simulink model "simulink_ODE_solved"  (R2023a)
settings: Solver=ode45  StartTime=0.0  StopTime=3000  RelTol=1e-3
settings Model: Creator=USER  LastModifiedBy=USER

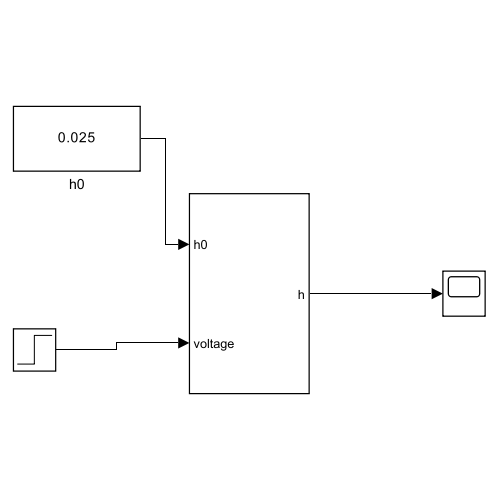
[thumbnail: Simulink's stored preview of the top-level diagram]
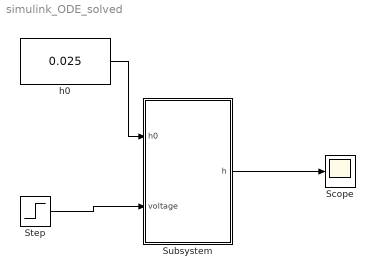
== system simulink_ODE_solved ==
  Scope : Scope
  Step : Step  Time=0  After=5  SampleTime=0.01
  Subsystem : Subsystem
  h0 : Constant  Value=0.025
  wires:
  h0/1 -> Subsystem/1(h0)
  Step/1 -> Subsystem/2(voltage)
  Subsystem/1(h) -> Scope/1

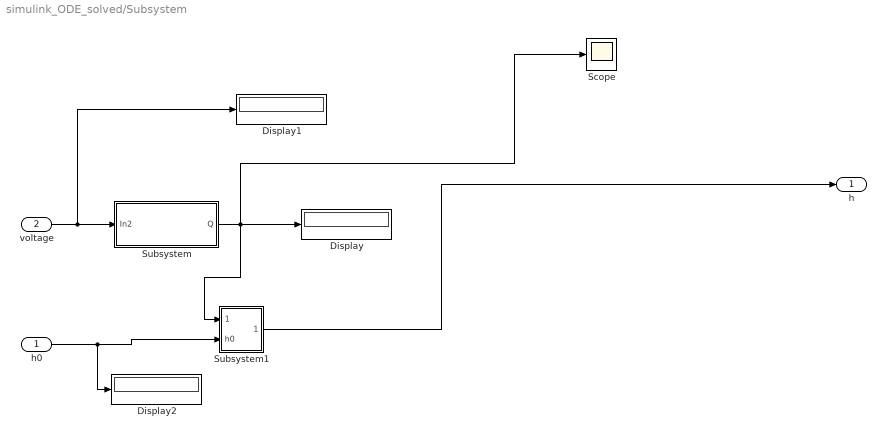
== system simulink_ODE_solved/Subsystem ==
  h0 : Inport
  voltage : Inport  Port=2
  Display : Display
  Display1 : Display
  Display2 : Display
  Scope : Scope
  Subsystem : Subsystem
  Subsystem1 : Subsystem
  h : Outport
  wires:
  Subsystem/1(Q) -> Scope/1, Subsystem1/1(In1), Display/1
  h0/1 -> Display2/1, Subsystem1/2(h0)
  Subsystem1/1(Out1) -> h/1
  voltage/1 -> Display1/1, Subsystem/1(In2)

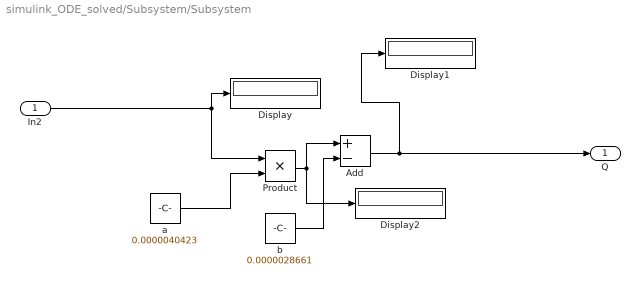
== system simulink_ODE_solved/Subsystem/Subsystem ==
  In2 : Inport
  Add : Sum  Inputs=+-
  Display : Display
  Display1 : Display
  Display2 : Display
  Product : Product
  a : Constant  Value=0.0000040423
  b : Constant  Value=0.0000028661
  Q : Outport
  wires:
  a/1 -> Product/2
  Product/1 -> Add/1, Display2/1
  b/1 -> Add/2
  Add/1 -> Display1/1, Q/1
  In2/1 -> Product/1, Display/1

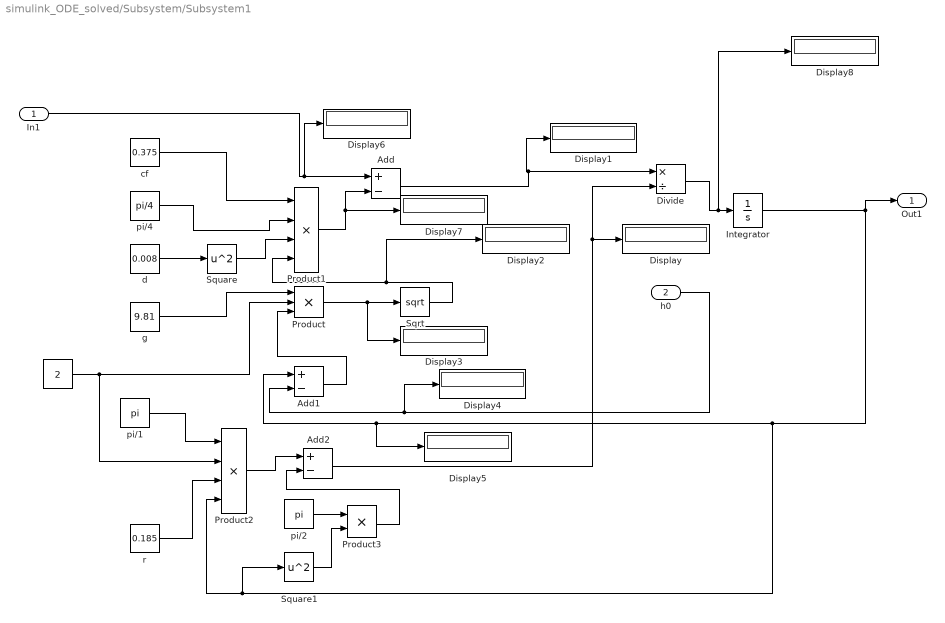
== system simulink_ODE_solved/Subsystem/Subsystem1 ==
  In1 : Inport
  h0 : Inport  Port=2
  " " : Constant  Value=2
  Add : Sum  Inputs=+-
  Add1 : Sum  Inputs=+-
  Add2 : Sum  Inputs=+-
  Display{,1..8} (9 alike) : Display
  Divide : Product  Inputs=*/
  Integrator : Integrator  InitialCondition=0.025
  Product : Product  Inputs=3
  Product1 : Product  Inputs=4
  Product2 : Product  Inputs=4
  Product3 : Product
  Sqrt : Sqrt
  Square : Math  Operator=square
  Square1 : Math  Operator=square
  cf : Constant  Value=0.375
  d : Constant  Value=0.008
  g : Constant  Value=9.81
  pi/1 : Constant  Value=pi
  pi/2 : Constant  Value=pi
  pi/4 : Constant  Value=pi/4
  r : Constant  Value=0.185
  Out1 : Outport
  wires:
  pi/1/1 -> Product2/1
  Add1/1 -> Product/3
  Product1/1 -> Display7/1, Add/2
  Divide/1 -> Display8/1, Integrator/1
  Product3/1 -> Add2/2
  " "/1 -> Product2/2, Product/2
  cf/1 -> Product1/1
  r/1 -> Product2/3
  Sqrt/1 -> Display2/1, Product1/4
  Square/1 -> Product1/3
  Product2/1 -> Add2/1
  pi/4/1 -> Product1/2
  h0/1 -> Display4/1, Add1/2
  g/1 -> Product/1
  d/1 -> Square/1
  Product/1 -> Display3/1, Sqrt/1
  Add/1 -> Divide/1, Display1/1
  Square1/1 -> Product3/2
  In1/1 -> Add/1, Display6/1
  pi/2/1 -> Product3/1
  Add2/1 -> Display/1, Divide/2
  Integrator/1 -> Out1/1, Product2/4, Square1/1, Display5/1, Add1/1
